simulink model "variant_workspace_Series_shunt_motor"  (R2024b)
settings: Solver=FixedStepDiscrete  StartTime=0.0  StopTime=0.6  RelTol=1e-3  EnableMultiTasking=on
values from neighbouring files (symbols this model uses):
  belt_thickness = 0.005    [variant_workspace.mat]
  radius = 0.113    [variant_workspace.mat]
settings Model: SimulationMode=external  ExtModeTrigDuration=8  Creator=admin
settings SolverCC: AlgebraicLoopSolver=TrustRegion  AutoInsertRateTranBlk=on
settings DataIOCC: ReturnWorkspaceOutputs=off
settings OptimizationCC: DefaultUnderspecifiedDataType=single  PassReuseOutputArgsAs=Individual arguments  MaxStackSize=512  EfficientTunableParamExpr=on
settings DebuggingCC: ParameterTunabilityLossMsg=error  UnconnectedInputMsg=warning  UnconnectedOutputMsg=warning  UnconnectedLineMsg=warning  ArithmeticOperatorsInVariantConditions=warning
settings HardwareCC: ProdBitPerChar=16  ProdBitPerInt=16  ProdBitPerPointer=32  ProdBitPerSizeT=32  ProdBitPerPtrDiffT=32  ProdLargestAtomicInteger=Integer  ProdLargestAtomicFloat=None  ProdWordSize=16  ProdLongLongMode=on  ProdHWDeviceType=Texas Instruments->C2000
settings ModelReferenceCC: EnableRefExpFcnMdlSchedulingChecks=on
settings SFSimCC: SimUseLocalCustomCode=off  MATLABDynamicMemAlloc=off  CustomCodeUndefinedFunction=UseInterfaceOnly
settings RTWCC: Description=Embedded Coder  SystemTargetFile=ert.tlc  HardwareBoard=TI Piccolo F2802x  GenCodeOnly=on  TemplateMakefile=ert_default_tmf  GenerateReport=on  RTWUseLocalCustomCode=off  Toolchain=Texas Instruments Code Composer Studio (C2000)  IncludeHyperlinkInReport=on  LaunchReport=on  GenerateTraceInfo=on  GenerateTraceReport=on  GenerateTraceReportSl=on  GenerateTraceReportSf=on  GenerateTraceReportEml=on  GPUComputeCapability=3.5
settings CodeAppCC: ForceParamTrailComments=on  IgnoreCustomStorageClasses=off  OperatorAnnotations=on  SimulinkDataObjDesc=on  SFDataObjDesc=on  MATLABFcnDesc=on  InsertBlockDesc=on  StateflowObjectComments=on  MATLABSourceComments=on
settings ERTTargetCC: CodeReplacementLibrary=TI C28x  SupportContinuousTime=on  ExtMode=on  ExtModeTransport=3  ExtModeMexArgs='127.0.0.1' 0 17725  InlinedParameterPlacement=Hierarchical  DynamicArrayContainerType=coder::array

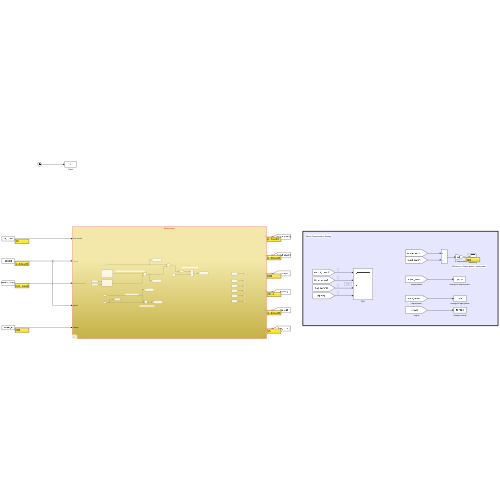
[thumbnail: Simulink's stored preview of the top-level diagram]
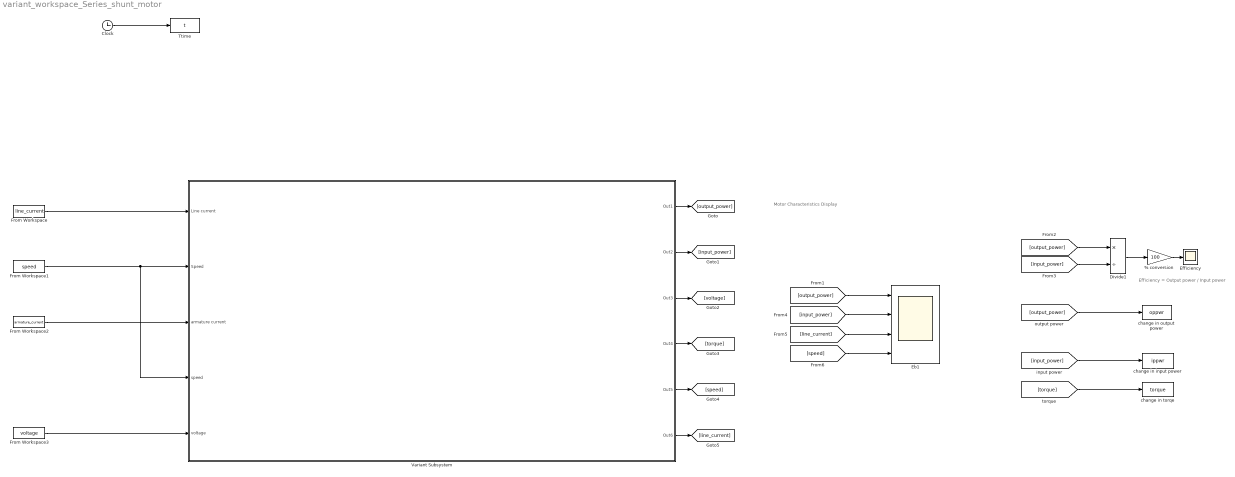
== system variant_workspace_Series_shunt_motor ==
  note: Efficiency = Output power / Input power
  note: Motor Characteristics Display
  % conversion : Gain  Gain=100
  Clock : Clock
  Divide1 : Product  Inputs=*/
  Eb1 : Scope  NumInputPorts=4
  "Efficiency " : Scope
  From Workspace : FromWorkspace  VariableName=line_current  SampleTime=0.1
  From Workspace1 : FromWorkspace  VariableName=speed  SampleTime=0.1
  From Workspace2 : FromWorkspace  VariableName=armature_current  SampleTime=-1
  From Workspace3 : FromWorkspace  VariableName=voltage  SampleTime=-1
  Ttime : ToWorkspace  VariableName=t  SampleTime=-1
  Variant Subsystem : Subsystem  Variant=on
  "change in input power " : ToWorkspace  VariableName=ippwr  SampleTime=-1
  change in output power : ToWorkspace  VariableName=oppwr  SampleTime=-1
  change in torqe : ToWorkspace  VariableName=torque  SampleTime=-1
  wires:
  Clock/1 -> Ttime/1
  [input_power] -> "change in input power "/1
  [output_power] -> change in output power/1
  [output_power] -> Divide1/1
  [input_power] -> Divide1/2
  [torque] -> change in torqe/1
  [output_power] -> Eb1/1
  [input_power] -> Eb1/2
  [line_current] -> Eb1/3
  [speed] -> Eb1/4
  % conversion/1 -> "Efficiency "/1
  Divide1/1 -> % conversion/1
  From Workspace/1 -> Variant Subsystem/1(Line current)
  From Workspace3/1 -> Variant Subsystem/5(voltage)
  From Workspace1/1 -> Variant Subsystem/4(speed), Variant Subsystem/2(Speed)
  From Workspace2/1 -> Variant Subsystem/3(armature current)
  Variant Subsystem/1(Out1) -> [output_power]
  Variant Subsystem/2(Out2) -> [input_power]
  Variant Subsystem/3(Out3) -> [voltage]
  Variant Subsystem/4(Out4) -> [torque]
  Variant Subsystem/5(Out5) -> [speed]
  Variant Subsystem/6(Out6) -> [line_current]

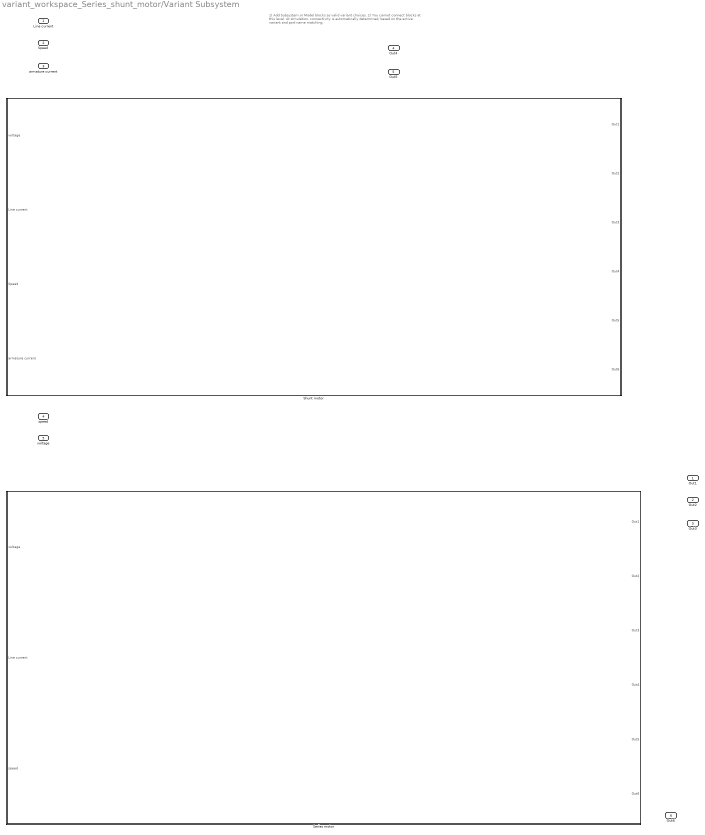
== system variant_workspace_Series_shunt_motor/Variant Subsystem ==
  note: 1) Add Subsystem or Model blocks as valid variant choices.
      | 2) You cannot connect blocks at this level. At simulation, connectivity is automatically
      | determined, based on the active variant and port name matching.
  Line current : Inport
  Speed : Inport  Port=2
  armature current : Inport  Port=3
  speed : Inport  Port=4
  voltage : Inport  Port=5
  Series motor : Subsystem  VariantControl=configuration == 2
  Shunt motor : Subsystem  VariantControl=configuration == 1
  Out1 : Outport
  Out2 : Outport  Port=2
  Out3 : Outport  Port=3
  Out4 : Outport  Port=4
  Out5 : Outport  Port=5
  Out6 : Outport  Port=6

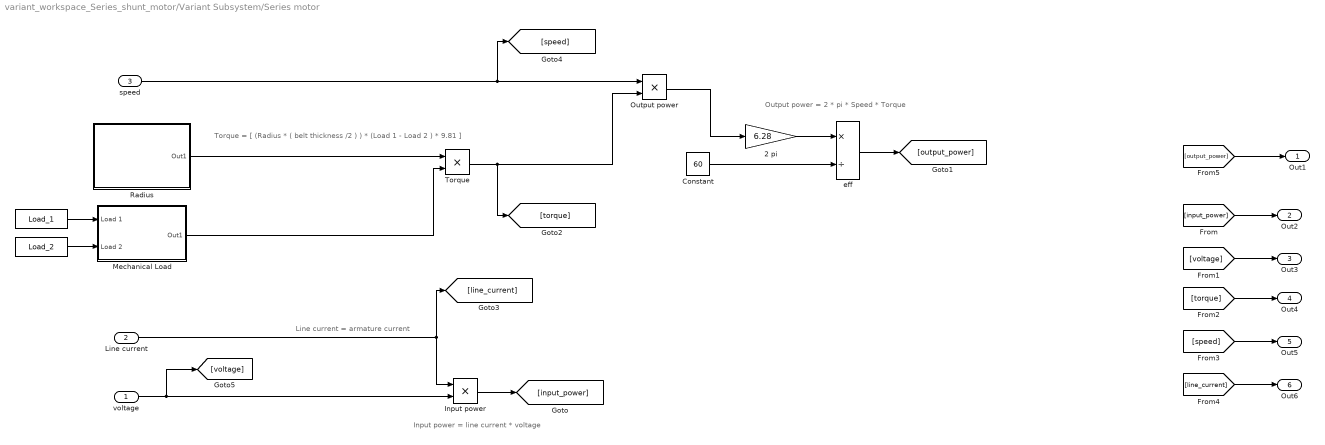
== system variant_workspace_Series_shunt_motor/Variant Subsystem/Series motor ==
  note: Input power = line current * voltage
  note: Line current = armature current
  note: Output power = 2 * pi * Speed * Torque
  note: Torque = [ (Radius * ( belt thickness /2 ) ) * (Load 1 - Load 2 ) * 9.81 ]
  voltage : Inport
  Line current : Inport  Port=2
  speed : Inport  Port=3
  " " : FromWorkspace  VariableName=Load_1  SampleTime=-1
  "  " : FromWorkspace  VariableName=Load_2  SampleTime=-1
  2 pi : Gain  Gain=6.28
  Constant : Constant  Value=60
  Input power : Product
  Mechanical Load : Subsystem
  Output power : Product
  Radius : Subsystem
  Torque : Product
  eff : Product  Inputs=*/
  Out1 : Outport
  Out2 : Outport  Port=2
  Out3 : Outport  Port=3
  Out4 : Outport  Port=4
  Out5 : Outport  Port=5
  Out6 : Outport  Port=6
  wires:
  Input power/1 -> [input_power]
  " "/1 -> Mechanical Load/1(Load 1)
  Torque/1 -> [torque], Output power/2
  2 pi/1 -> eff/1
  Output power/1 -> 2 pi/1
  speed/1 -> [speed], Output power/1
  Mechanical Load/1(Out1) -> Torque/2
  "  "/1 -> Mechanical Load/2(Load 2)
  Radius/1(Out1) -> Torque/1
  voltage/1 -> [voltage], Input power/2
  Line current/1 -> [line_current], Input power/1
  eff/1 -> [output_power]
  Constant/1 -> eff/2
  [voltage] -> Out3/1
  [torque] -> Out4/1
  [speed] -> Out5/1
  [line_current] -> Out6/1
  [output_power] -> Out1/1
  [input_power] -> Out2/1

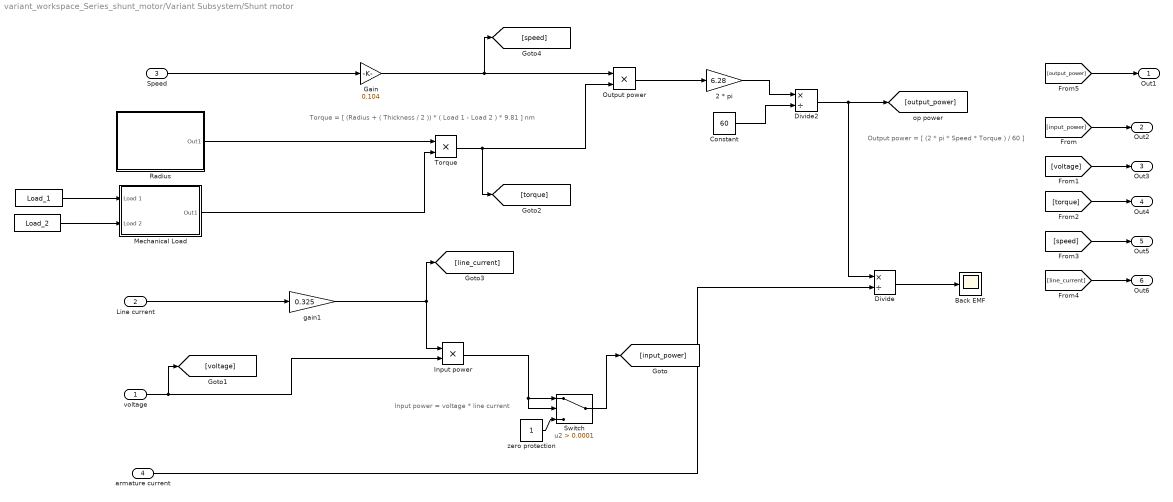
== system variant_workspace_Series_shunt_motor/Variant Subsystem/Shunt motor ==
  note: Input power = voltage * line current
  note: Output power = [ (2 * pi * Speed * Torque ) / 60 ]
  note: Torque = [ (Radius + ( Thickness / 2 )) * ( Load 1 - Load 2 ) * 9.81 ] nm
  voltage : Inport
  Line current : Inport  Port=2
  Speed : Inport  Port=3
  armature current : Inport  Port=4
  " " : FromWorkspace  VariableName=Load_1  SampleTime=-1
  "  " : FromWorkspace  VariableName=Load_2  SampleTime=-1
  2 * pi : Gain  Gain=6.28
  Back EMF : Scope
  Constant : Constant  Value=60
  Divide : Product  Inputs=*/
  Divide2 : Product  Inputs=*/
  Gain : Gain  Gain=0.104
  Input power : Product
  Mechanical Load : Subsystem
  Output power : Product
  Radius : Subsystem
  Switch : Switch  Criteria=u2 > Threshold  Threshold=0.0001  SaturateOnIntegerOverflow=off  InputSameDT=off
  Torque : Product
  gain1 : Gain  Gain=0.325
  zero protection : Constant
  Out1 : Outport
  Out2 : Outport  Port=2
  Out3 : Outport  Port=3
  Out4 : Outport  Port=4
  Out5 : Outport  Port=5
  Out6 : Outport  Port=6
  wires:
  "  "/1 -> Mechanical Load/2(Load 2)
  Mechanical Load/1(Out1) -> Torque/2
  " "/1 -> Mechanical Load/1(Load 1)
  gain1/1 -> [line_current], Input power/1
  2 * pi/1 -> Divide2/1
  Divide2/1 -> Divide/1, [output_power]
  Line current/1 -> gain1/1
  Constant/1 -> Divide2/2
  Torque/1 -> [torque], Output power/2
  Output power/1 -> 2 * pi/1
  Divide/1 -> Back EMF/1
  armature current/1 -> Divide/2
  Radius/1(Out1) -> Torque/1
  [input_power] -> Out2/1
  [voltage] -> Out3/1
  voltage/1 -> [voltage], Input power/2
  [speed] -> Out5/1
  [torque] -> Out4/1
  [line_current] -> Out6/1
  [output_power] -> Out1/1
  Switch/1 -> [input_power]
  Input power/1 -> Switch/1, Switch/2
  zero protection/1 -> Switch/3
  Speed/1 -> Gain/1
  Gain/1 -> [speed], Output power/1

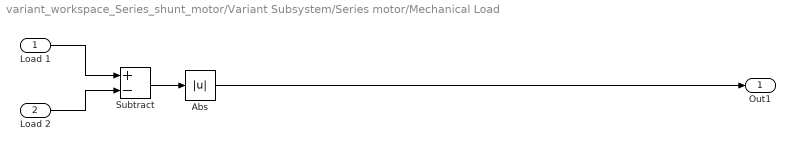
== system variant_workspace_Series_shunt_motor/Variant Subsystem/Series motor/Mechanical Load ==
  Load 1 : Inport
  Load 2 : Inport  Port=2
  Abs : Abs  SaturateOnIntegerOverflow=off
  Subtract : Sum  Inputs=+-
  Out1 : Outport
  wires:
  Load 1/1 -> Subtract/1
  Load 2/1 -> Subtract/2
  Abs/1 -> Out1/1
  Subtract/1 -> Abs/1

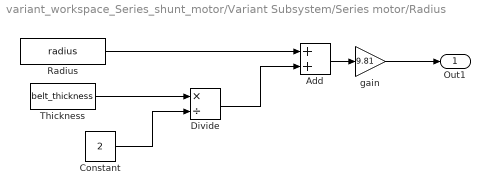
== system variant_workspace_Series_shunt_motor/Variant Subsystem/Series motor/Radius ==
  Add : Sum
  Constant : Constant  Value=2
  Divide : Product  Inputs=*/
  Radius : Constant  Value=radius  SampleTime=-1
  Thickness : Constant  Value=belt_thickness  SampleTime=-1
  gain : Gain  Gain=9.81
  Out1 : Outport
  wires:
  Radius/1 -> Add/1
  Add/1 -> gain/1
  gain/1 -> Out1/1
  Thickness/1 -> Divide/1
  Divide/1 -> Add/2
  Constant/1 -> Divide/2

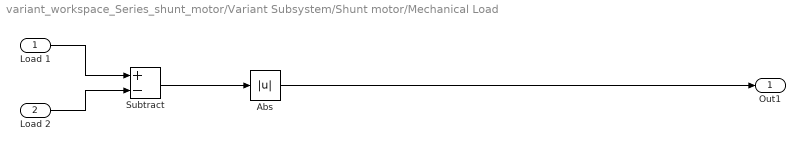
== system variant_workspace_Series_shunt_motor/Variant Subsystem/Shunt motor/Mechanical Load ==
  Load 1 : Inport
  Load 2 : Inport  Port=2
  Abs : Abs  SaturateOnIntegerOverflow=off
  Subtract : Sum  Inputs=+-
  Out1 : Outport
  wires:
  Load 1/1 -> Subtract/1
  Load 2/1 -> Subtract/2
  Abs/1 -> Out1/1
  Subtract/1 -> Abs/1

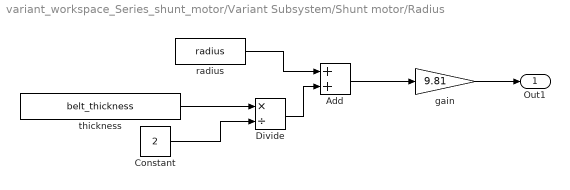
== system variant_workspace_Series_shunt_motor/Variant Subsystem/Shunt motor/Radius ==
  Add : Sum
  Constant : Constant  Value=2
  Divide : Product  Inputs=*/
  gain : Gain  Gain=9.81
  radius : Constant  Value=radius
  thickness : Constant  Value=belt_thickness
  Out1 : Outport
  wires:
  radius/1 -> Add/1
  Add/1 -> gain/1
  gain/1 -> Out1/1
  thickness/1 -> Divide/1
  Divide/1 -> Add/2
  Constant/1 -> Divide/2
